simulink model "ann_crystallizer_model_for_training"  (R2024a)
settings: Solver=VariableStepAuto  StartTime=0.0  StopTime=10.0  RelTol=1e-3
settings Model: Creator=Ranjeet  LastModifiedBy=Ranjeet

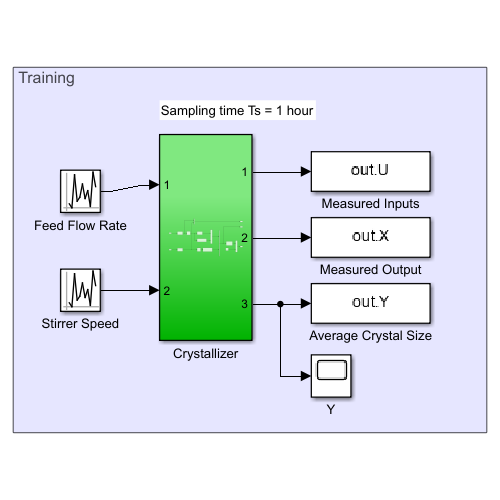
[thumbnail: Simulink's stored preview of the top-level diagram]
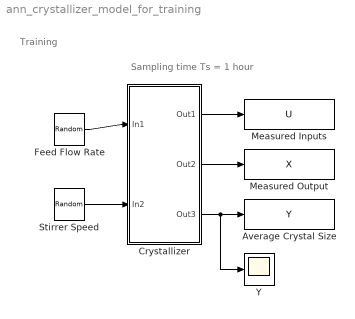
== system ann_crystallizer_model_for_training ==
  note: Training
  note: Sampling time Ts = 1 hour
  Average Crystal Size : ToWorkspace  VariableName=Y  SampleTime=1
  Crystallizer : Subsystem
  Feed Flow Rate : UniformRandomNumber  Minimum=-1.2  Maximum=1.2  SampleTime=1
  Measured Inputs : ToWorkspace  VariableName=U  SampleTime=1
  Measured Output : ToWorkspace  VariableName=X  SampleTime=1
  Stirrer Speed : UniformRandomNumber  Minimum=-1.5  Maximum=1.5  SampleTime=1
  Y : Scope
  wires:
  Feed Flow Rate/1 -> Crystallizer/1(In1)
  Crystallizer/2(Out2) -> Measured Output/1
  Crystallizer/1(Out1) -> Measured Inputs/1
  Stirrer Speed/1 -> Crystallizer/2(In2)
  Crystallizer/3(Out3) -> Y/1, Average Crystal Size/1

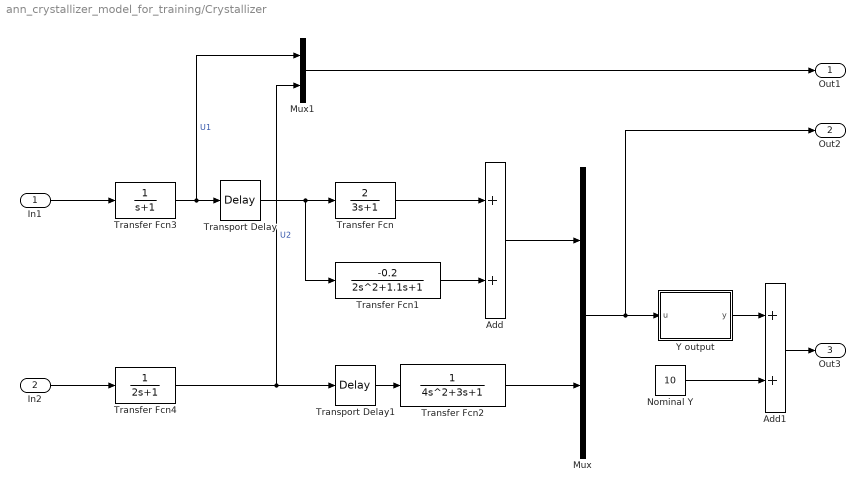
== system ann_crystallizer_model_for_training/Crystallizer ==
  In1 : Inport
  In2 : Inport  Port=2
  Add : Sum
  Add1 : Sum
  Mux : Mux  Inputs=2
  Mux1 : Mux  Inputs=2
  Nominal Y : Constant  Value=10
  Transfer Fcn : TransferFcn  Numerator=[2]  Denominator=[3 1]
  Transfer Fcn1 : TransferFcn  Numerator=[-0.2]  Denominator="[2  1.1  1]"
  Transfer Fcn2 : TransferFcn  Denominator="[4  3   1]"
  Transfer Fcn3 : TransferFcn  Denominator=[1 1]
  Transfer Fcn4 : TransferFcn  Denominator=[2 1]
  Transport Delay : TransportDelay
  Transport Delay1 : TransportDelay
  Y output : MATLAB Function  TreatAsAtomicUnit=on
  Out1 : Outport
  Out2 : Outport  Port=2
  Out3 : Outport  Port=3
  wires:
  Transfer Fcn2/1 -> Mux/2
  Transport Delay/1 -> Transfer Fcn/1, Transfer Fcn1/1
  Y output/1(y) -> Add1/1
  Nominal Y/1 -> Add1/2
  Transfer Fcn/1 -> Add/1
  Transfer Fcn3/1 -> Transport Delay/1, Mux1/1  "U1"
  Transport Delay1/1 -> Transfer Fcn2/1
  Transfer Fcn4/1 -> Mux1/2, Transport Delay1/1  "U2"
  Mux/1 -> Out2/1, Y output/1(u)
  Add/1 -> Mux/1
  Add1/1 -> Out3/1
  In2/1 -> Transfer Fcn4/1
  Transfer Fcn1/1 -> Add/2
  In1/1 -> Transfer Fcn3/1
  Mux1/1 -> Out1/1

== matlab function ann_crystallizer_model_for_training/Crystallizer/Y output ==
  data: u input; y output
function y = fcn(u)

y = 0.8*u(1) + 1.3*u(2) + 1.1*(u(1)^2) - 1.9*(u(2)^2) + 0.6*u(1)*u(2);
